simulink library "standardBlocks_lib"  (R2018b)
settings: Solver=VariableStepAuto  StartTime=0.0  StopTime=10.0  RelTol=1e-3
undefined symbols (not defined in the file or in its folder): DiscIntNeverNeededParam, fswParams, simParams
libraries: simulink x1
settings Model: Creator=colem  LastModifiedBy=colem

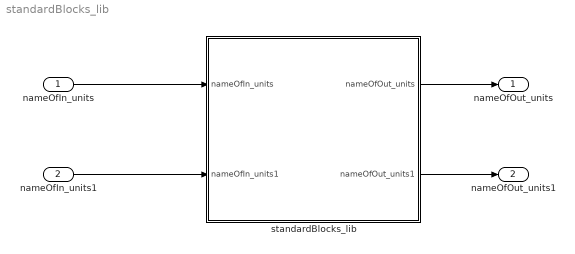
== system standardBlocks_lib ==
  nameOfIn_units : Inport
  nameOfIn_units1 : Inport  Port=2
  standardBlocks_lib : Subsystem
  nameOfOut_units : Outport
  nameOfOut_units1 : Outport  Port=2
  wires:
  nameOfIn_units/1 -> standardBlocks_lib/1(nameOfIn_units)
  nameOfIn_units1/1 -> standardBlocks_lib/2(nameOfIn_units1)
  standardBlocks_lib/1(nameOfOut_units) -> nameOfOut_units/1
  standardBlocks_lib/2(nameOfOut_units1) -> nameOfOut_units1/1

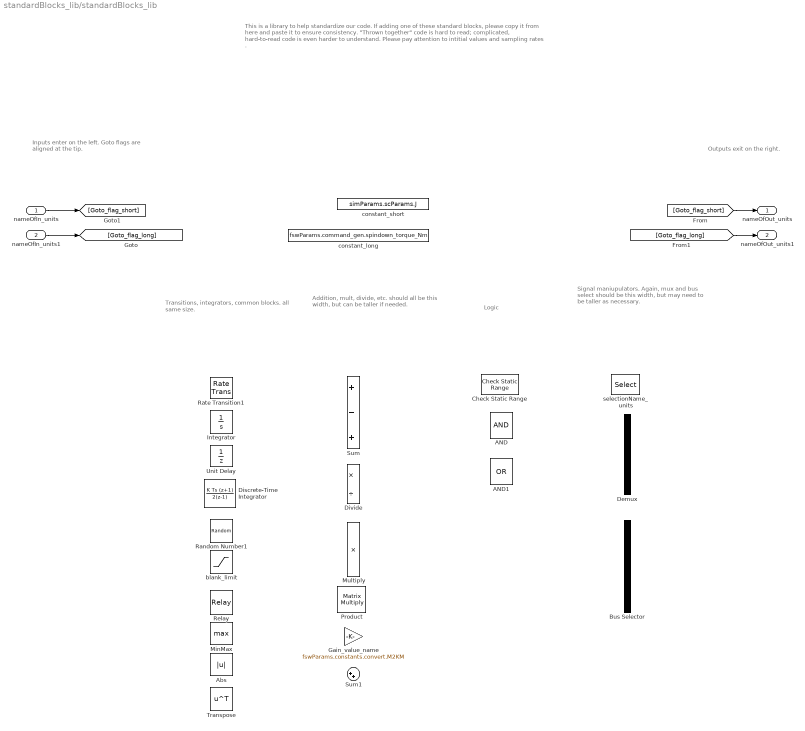
== system standardBlocks_lib/standardBlocks_lib ==
  note: This is a library to help standardize our code. If adding one of these standard blocks, please copy it from here and paste it to ensure consistency. "Thrown together" code is hard to read; complicated, hard-to-read code is even harder to understand. Please pay attention to intitial values and sampling rates .
  note: Inputs enter on the left. Goto flags are aligned at the tip.
  note: Outputs exit on the right.
  note: Transitions, integrators, common blocks. all same size.
  note: Addition, mult, divide, etc. should all be this width, but can be taller if needed.
  note: Logic
  note: Signal maniupulators. Again, mux and bus select should be this width, but may need to be taller as necessary.
  nameOfIn_units : Inport
  nameOfIn_units1 : Inport  Port=2
  AND : Logic  AllPortsSameDT=off  OutDataTypeStr=boolean
  AND1 : Logic  Operator=OR  AllPortsSameDT=off  OutDataTypeStr=boolean
  Abs : Abs
  Bus Selector : BusSelector  OutputSignals=r_eci_km,v_eci_km,q_body,w_body_radps
  Check Static Range : simulink/Model Verification/Check  Static Range  Description=-simParams.actuators.rwa.max_RPM < u < simParams.actuators.rwa.max_RPM  max=simParams.actuators.rwa.max_RPM  max_included=off  min=-simParams.actuators.rwa.max_RPM  min_included=off  enabled=on  stopWhenAssertionFail=off  export=on  icon=graphic
      settings: SourceProductName=Simulink  SourceProductBaseCode=SL
  Demux : Demux  Outputs=[1 1]
  Discrete-Time Integrator : DiscreteIntegrator  IntegratorMethod=Integration: Trapezoidal  InitialCondition=simParams.initialConditions.v0  SampleTime=-1  ICPrevOutput=DiscIntNeverNeededParam  ICPrevScaledInput=DiscIntNeverNeededParam
  Divide : Product  Inputs=*/
  Gain_value_name : Gain  Gain=fswParams.constants.convert.M2KM
  Integrator : Integrator  InitialCondition=simParams.initialConditions.v0
  MinMax : MinMax  Function=max
  Multiply : Product  Inputs=3
  Product : Product  Multiplication=Matrix(*)
  Random Number1 : RandomNumber  Variance=simParams.actuators.rwa.rpm_variance  Seed=1  SampleTime=simParams.sample_time_s
  Rate Transition1 : RateTransition  OutPortSampleTime=simParams.sample_time_s
  Relay : Relay  OnSwitchValue=fswParams.mode_select.body_rate_threshold_max  OffSwitchValue=fswParams.mode_select.body_rate_threshold_min
  Sum : Sum  Inputs=+-+
  Sum1 : Sum  Inputs=|++
  Transpose : Math  Operator=transpose  SaturateOnIntegerOverflow=on
  Unit Delay : UnitDelay  InitialCondition=[1;1;1;1;1;1;1;1;1;0;0;simParams.actuators.rwa.ic.rpm]  SampleTime=simParams.sample_time_s
  blank_limit : Saturate  UpperLimit=simParams.sensors.sun_sensor.range_deg  LowerLimit=-simParams.sensors.sun_sensor.range_deg
  constant_long : Constant  Value=fswParams.command_gen.spindown_torque_Nm  SampleTime=fswParams.sample_time_s
  constant_short : Constant  Value=simParams.scParams.J  SampleTime=fswParams.sample_time_s
  selectionName_units : Selector  InputPortWidth=13  IndexOptions=Index vector (dialog)  Indices=fswParams.constants.id_r  OutputSizes=1
  nameOfOut_units : Outport
  nameOfOut_units1 : Outport  Port=2
  wires:
  nameOfIn_units1/1 -> [Goto_flag_long]
  [Goto_flag_short] -> nameOfOut_units/1
  [Goto_flag_long] -> nameOfOut_units1/1
  nameOfIn_units/1 -> [Goto_flag_short]
